simulink subsystem "startOLAESolSelector"  (R2021a)
settings: Solver=VariableStepAuto  StartTime=0.0  StopTime=10.0  RelTol=1e-3
libraries: sharedutil x2, aerolibutil x2
settings Model: Creator=noraw  LastModifiedBy=noraw

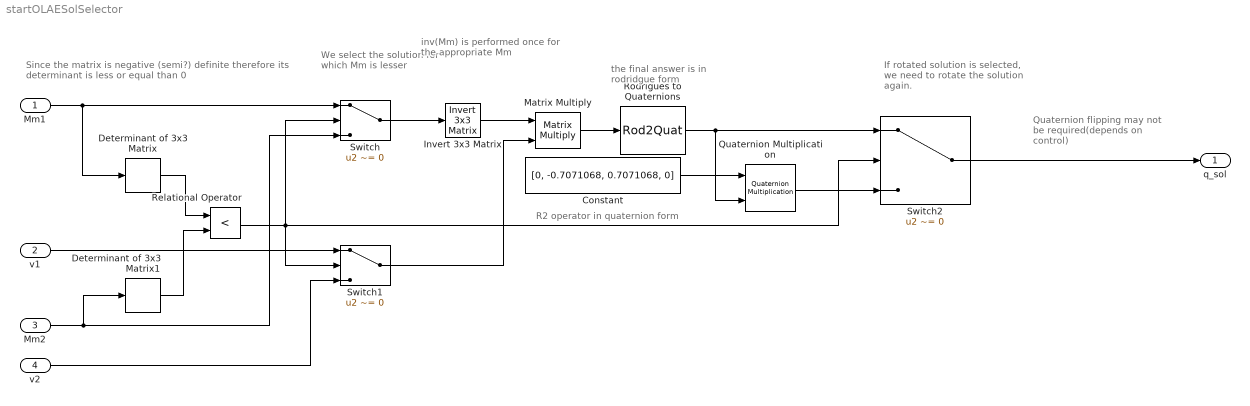
== system startOLAESolSelector ==
  note: Since the matrix is negative (semi?) definite therefore
      | its determinant is less or equal than 0
  note: R2 operator in quaternion form
  note: We select the solution for
      | which Mm is lesser
  note: inv(Mm) is performed once for the appropriate Mm
  note: the final answer is in rodridgue form
  note: If rotated solution is selected, we need to rotate the solution again.
  note: Quaternion flipping may not be required(depends on control)
  Mm1 : Inport
  v1 : Inport  Port=2
  Mm2 : Inport  Port=3
  v2 : Inport  Port=4
  Constant : Constant  Value=[0, -0.7071068, 0.7071068, 0]
  Determinant of 3x3 Matrix : sharedutil/Determinant of 3x3 Matrix  aMode=aMode
      settings: SourceProductBaseCode=AE,PW,DR,MT,UV,VE
  Determinant of 3x3 Matrix1 : sharedutil/Determinant of 3x3 Matrix  aMode=aMode
      settings: SourceProductBaseCode=AE,PW,DR,MT,UV,VE
  Invert 3x3 Matrix : aerolibutil/Invert  3x3 Matrix
  Matrix Multiply : Product  Multiplication=Matrix(*)
  Quaternion Multiplication : aerolibutil/Quaternion Multiplication
  Relational Operator : RelationalOperator  Operator=<  OutDataTypeStr=boolean  RndMeth=Simplest
  Rodrigues to Quaternions : Rod2Quat
  Switch : Switch  Criteria=u2 ~= 0  ZeroCross=off
  Switch1 : Switch  Criteria=u2 ~= 0  ZeroCross=off
  Switch2 : Switch  Criteria=u2 ~= 0
  q_sol : Outport
  wires:
  Determinant of 3x3 Matrix1/1 -> Relational Operator/2
  Mm2/1 -> Determinant of 3x3 Matrix1/1, Switch/3
  Switch/1 -> Invert 3x3 Matrix/1
  Rodrigues to Quaternions/1 -> Switch2/1, Quaternion Multiplication/2
  Relational Operator/1 -> Switch/2, Switch2/2, Switch1/2
  Determinant of 3x3 Matrix/1 -> Relational Operator/1
  Mm1/1 -> Determinant of 3x3 Matrix/1, Switch/1
  Matrix Multiply/1 -> Rodrigues to Quaternions/1
  Quaternion Multiplication/1 -> Switch2/3
  Switch1/1 -> Matrix Multiply/2
  Invert 3x3 Matrix/1 -> Matrix Multiply/1
  v2/1 -> Switch1/3
  v1/1 -> Switch1/1
  Switch2/1 -> q_sol/1
  Constant/1 -> Quaternion Multiplication/1
